simulink library "CTRL_SPECCTRL_FB_STRAT2"  (R2024b)
settings: Solver=VariableStepAuto  StartTime=0.0  StopTime=10.0  RelTol=1e-3
settings Model: Creator=blatak  LastModifiedBy=blatak

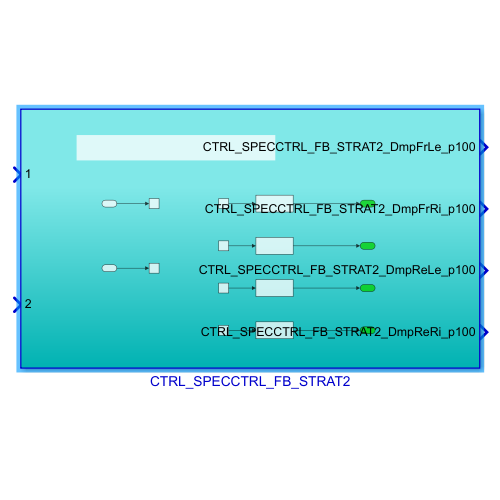
[thumbnail: Simulink's stored preview of the top-level diagram]
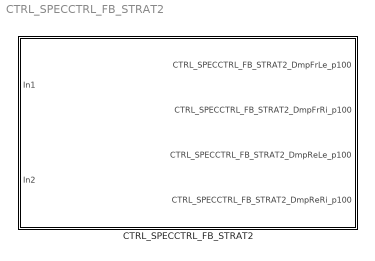
== system CTRL_SPECCTRL_FB_STRAT2 ==
  CTRL_SPECCTRL_FB_STRAT2 : Subsystem

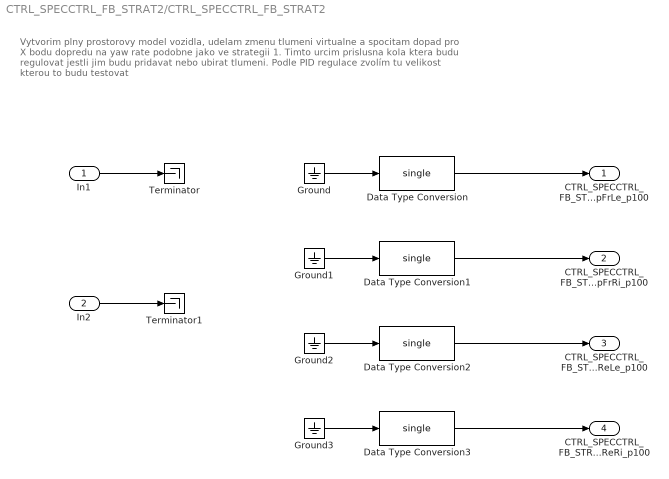
== system CTRL_SPECCTRL_FB_STRAT2/CTRL_SPECCTRL_FB_STRAT2 ==
  note: Vytvorim plny prostorovy model vozidla, udelam zmenu tlumeni virtualne a spocitam dopad pro X bodu dopredu na yaw rate podobne jako ve strategii 1. Timto urcim prislusna kola ktera budu regulovat jestli jim budu pridavat nebo ubirat tlumeni. Podle PID regulace zvolím tu velikost kterou to budu testovat
  In1 : Inport
  In2 : Inport  Port=2
  Data Type Conversion{,1..3} (4 alike) : DataTypeConversion  OutDataTypeStr=single  SaturateOnIntegerOverflow=off  RndMeth=Floor
  Ground{,1..3} (4 alike) : Ground
  Terminator : Terminator
  Terminator1 : Terminator
  CTRL_SPECCTRL_FB_STRAT2_DmpFrLe_p100 : Outport
  CTRL_SPECCTRL_FB_STRAT2_DmpFrRi_p100 : Outport  Port=2
  CTRL_SPECCTRL_FB_STRAT2_DmpReLe_p100 : Outport  Port=3
  CTRL_SPECCTRL_FB_STRAT2_DmpReRi_p100 : Outport  Port=4
  wires:
  In1/1 -> Terminator/1
  In2/1 -> Terminator1/1
  Ground/1 -> Data Type Conversion/1
  Data Type Conversion/1 -> CTRL_SPECCTRL_FB_STRAT2_DmpFrLe_p100/1
  Ground1/1 -> Data Type Conversion1/1
  Ground2/1 -> Data Type Conversion2/1
  Ground3/1 -> Data Type Conversion3/1
  Data Type Conversion1/1 -> CTRL_SPECCTRL_FB_STRAT2_DmpFrRi_p100/1
  Data Type Conversion2/1 -> CTRL_SPECCTRL_FB_STRAT2_DmpReLe_p100/1
  Data Type Conversion3/1 -> CTRL_SPECCTRL_FB_STRAT2_DmpReRi_p100/1
